simulink subsystem "Mean_Subsystem"  (R2025b)
settings: Solver=VariableStepAuto  StartTime=0.0  StopTime=10.0  RelTol=1e-3
model mask{f=60, Ncycles=1, InitialValue=0}
  mask prompts: f "Fundamental frequency (Hz)"; InitialValue "Initial mean output"
values from neighbouring files (symbols this model uses):
  InitialValue = 0    [mean_init.m]
  T = Ncycles / f    [mean_init.m]
libraries: simulink x1
settings Model: Creator=Murl0  LastModifiedBy=Murl0

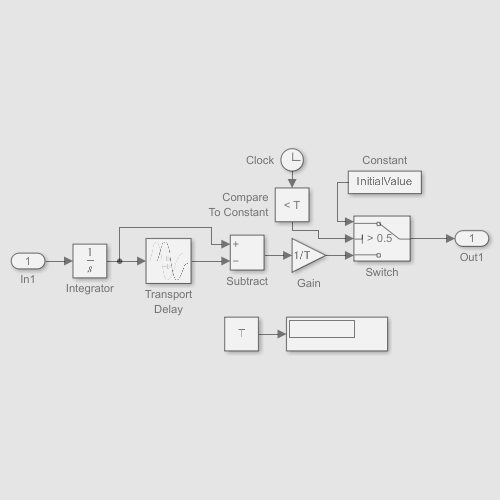
[thumbnail: Simulink's stored preview of the top-level diagram]
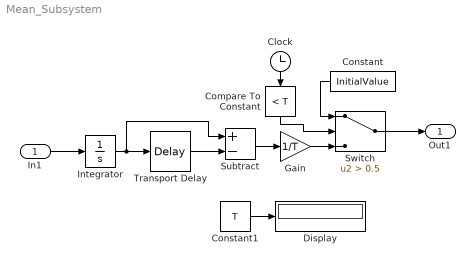
== system Mean_Subsystem ==
  In1 : Inport
  Clock : Clock
  Compare To Constant : simulink/Logic and Bit Operations/Compare To Constant  relop=<  const=T  OutDataTypeStr=boolean
  Constant : Constant  Value=InitialValue
  Constant1 : Constant  Value=T
  Display : Display
  Gain : Gain  Gain=1/T
  Integrator : Integrator
  Subtract : Sum  Inputs=+-
  Switch : Switch  Criteria=u2 > Threshold  Threshold=0.5  SaturateOnIntegerOverflow=off  InputSameDT=off
  Transport Delay : TransportDelay  DelayTime=T
  Out1 : Outport
  wires:
  Transport Delay/1 -> Subtract/2
  Switch/1 -> Out1/1
  In1/1 -> Integrator/1
  Integrator/1 -> Subtract/1, Transport Delay/1
  Gain/1 -> Switch/3
  Subtract/1 -> Gain/1
  Clock/1 -> Compare To Constant/1
  Constant/1 -> Switch/1
  Compare To Constant/1 -> Switch/2
  Constant1/1 -> Display/1
